simulink model "Spunto3"  (R2022a)
settings: Solver=VariableStepAuto  StartTime=0.0  StopTime=30  RelTol=1e-3
settings Model: Creator=bryan  LastModifiedBy=bryan

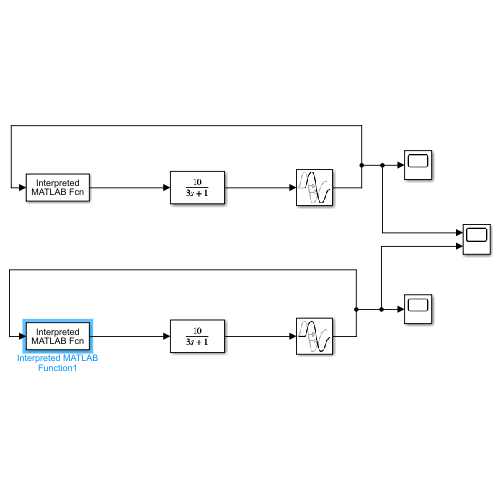
[thumbnail: Simulink's stored preview of the top-level diagram]
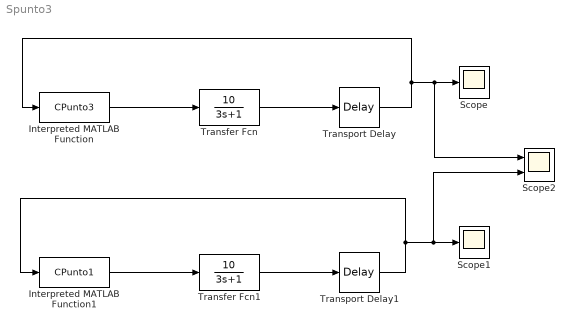
== system Spunto3 ==
  Interpreted MATLAB Function : MATLABFcn  MATLABFcn=CPunto3
  Interpreted MATLAB Function1 : MATLABFcn  MATLABFcn=CPunto1
  Scope : Scope
  Scope1 : Scope
  Scope2 : Scope  NumInputPorts=2
  Transfer Fcn : TransferFcn  Numerator=[10]  Denominator=[3 1]
  Transfer Fcn1 : TransferFcn  Numerator=[10]  Denominator=[3 1]
  Transport Delay : TransportDelay  DelayTime=0.2
  Transport Delay1 : TransportDelay  DelayTime=0.2
  wires:
  Interpreted MATLAB Function/1 -> Transfer Fcn/1
  Transfer Fcn/1 -> Transport Delay/1
  Transport Delay/1 -> Scope2/1, Scope/1, Interpreted MATLAB Function/1
  Transfer Fcn1/1 -> Transport Delay1/1
  Transport Delay1/1 -> Interpreted MATLAB Function1/1, Scope2/2, Scope1/1
  Interpreted MATLAB Function1/1 -> Transfer Fcn1/1
